simulink model "SCR_SiLS_R4_D102_test1"  (R2023a)
settings: Solver=VariableStepAuto  StartTime=0.0  StopTime=T_sim_end  RelTol=1e-3
model workspace (MAT data in the model file):
  ConnVar.ipAddress = '192.168.0.153'
  ConnVar.user = 'M1'
  ConnVar.pwd = [145 145 158 146 151 156 158 157]
  ConnVar.targetHandle = 0
libraries: M1SWBlocks x4
(part 1 of 2)
settings Model: Creator=CHSE  LastModifiedBy=gione
settings DebuggingCC: UnconnectedInputMsg=warning  UnconnectedOutputMsg=warning  UnconnectedLineMsg=warning
settings ModelReferenceCC: EnableRefExpFcnMdlSchedulingChecks=on
settings RTWCC: DLArmComputeVersion=19.05

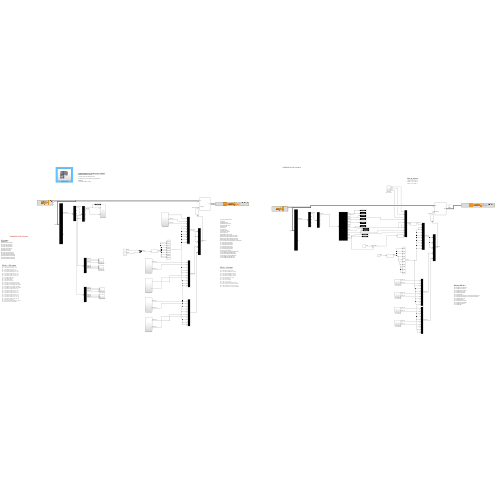
[thumbnail: Simulink's stored preview of the top-level diagram]
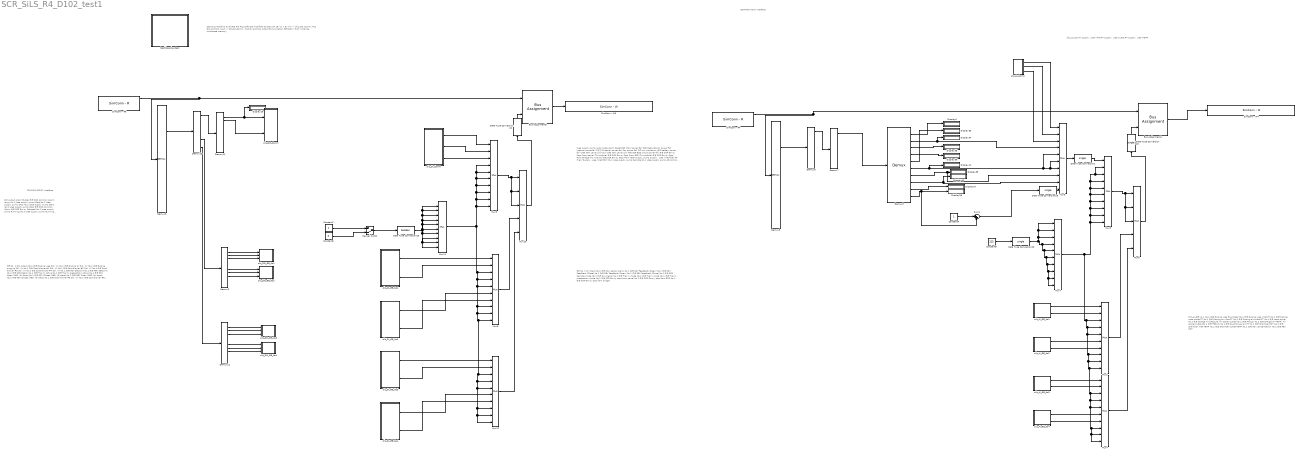
== system SCR_SiLS_R4_D102_test1 ==
  note: GE No. 1 DI intput
      |
      | No.1 G/E NOx sensor Alarm
      |
      | No.1 G/E RSV Feedback (Open)
      |
      | No.1 G/E RSV Feedback (Close)
      |
      | No.1 G/E RBV Feedback (Open)
      |
      | No.1 G/E RBV Feedback (Close)
      |
      | No.1 G/E SCR Remote mode
      |
      | No.1 G/E Run signal
      |
      | No.1 G/E Tier III mode
      |
      | No.1 G/E Tier II mode
      |
      | No.1 G/E Tier III preparation mode
      |
      | No.1 G/E SCR Em'cy stop from panel
      |
      | No.1 G/E SCR Emc'y stop from ECR
      |
      | No.1 G/E SCR Em'cy stop from bridge
  note: GE No. 1 DO output
      |
      | No.1 G/E Dosing urea Sol. VV
      |
      | No.1 G/E Dosing air Sol. VV
      |
      | No.1 G/E Dosing purging Sol. VV
      |
      | No.1 G/E Soot blower #1 Sol. VV
      |
      | No.1 G/E Soot blower #2 Sol. VV
      |
      | No.1 G/E Soot blower #3 Sol. VV
      |
      | No.1 G/E Soot blower #4 Sol. VV
      |
      | No.1 G/E RSV Setpoint
      |
      | No.1 G/E RBV Setpoint
      |
      | No.1 G/E SCR Ready
      |
      | No.1 G/E Tier III Active
      |
      | No.1 G/E Tier III preparation Active
      |
      | No.1 G/E RSV Open (ABS, NK class)
      |
      | No.1 G/E RSV Closed (ABS, NK class)
      |
      | No.1 G/E RBV Open (ABS, NK class)
      |
      | No.1 G/E RBV Closed (ABS, NK class)
      |
      | No.1 G/E Soot blower #5 Sol. VV
      |
      | No.1 G/E Soot blower #6 Sol. VV
      |
      | No.1 G/E Soot blower #7 Sol. VV
      |
      | No.1 G/E Soot blower #8 Sol. VV
      |
      | No.1 G/E Soot blower #9 Sol. VV
      |
      | No.1 G/E Soot blower #10 Sol. VV
      |
      | No.1 G/E Soot blower #11 Sol. VV
      |
      | No.1 G/E Soot blower #12 Sol. VV
      |
      | No.1 G/E Tier III Transfer
      |
      | No.1 SCR both bypass valve not open
      |
      | No.# G/E Common Shutdown
  note: DO output
      | Alarm Buzzer
      |
      | G/E SCR common alarm lamp
      |
      | No.1 Urea supply pump Start
      |
      | No.1 Urea supply pump Stop
      |
      | No.2 Urea supply pump Start
      |
      | No.2 Urea supply pump Stop
      |
      | G/E SCR common Alarm
      |
      | G/E SCR Em'cy Stopped
      |
      | No.1 Urea supply pump Running
      |
      | No.2 Urea supply pump Running
      |
      | No.1 G/E SCR Common Alarm lamp
      |
      | No.2 G/E SCR Common Alarm lamp
      |
      | No.3 G/E SCR Common Alarm lamp
      |
      | No.4 G/E SCR Common Alarm lamp
      |
      | ​
      |
      | ​
  note: Urea supply pump Auto mode
      |
      | Alarm Reset
      |
      | SCR Main power fail
      |
      | SCR Redundancy power fail
      |
      | Internal power fail(삭제됨)
      |
      | External power fail
      |
      | Fan power fail
      |
      | DC low insulation
      |
      | UPS battery power fail
      |
      | Urea tank Level Low-Low
      |
      | Urea tank Level Low
      |
      | G/E SCR ESD circuit power fail
      |
      | G/E SCR Em'cy Stop From panel (To module)
      |
      | G/E SCR Em'cy Stop From ECR (To module)
      |
      | G/E SCR Em'cy Stop From Bridge (To module)
      |
      | G/E SCR Em'cy Stop From Near Supply pump
      |
      | Supply, urea inlet filter dP High (Supply, urea inlet PDS)
      |
      | No.1 Urea supply pump Remote
      |
      | No.1 Urea supply pump Abnormal
      |
      | No.1 Urea supply pump Running
      |
      | No.2 Urea supply pump Remote
      |
      | No.2 Urea supply pump Abnormal
      |
      | No.2 Urea supply pump Running
      |
      | G/E Low Sulfur fuel supplied
      |
      | Urea tank drip tray Level High-High (ABS class)
      |
      | Urea tank TEMP High-High (ABS class)
      |
      | Urea tank Level High (ABS, BV, NK class)
      |
      | Urea tank drip tray Level High (ABS class)
      |
      | Urea tank TEMP Low (ABS, NK class)
      |
      | Urea tank TEMP High (ABS, NK class)
      |
      | ​
      |
      | ​
  note: COMMON DO/DI Interface
  note: SCR SiLS Model to evaluate the PLC software
      | modified at 2024.04.18. by Y.B. Kim
      |
      | -> Sils_DO_Comm: PLC DO and Sils input
      | -> Sils_DI_Comm : PLC DI and Sils output for simulation
      |
      | REMARK!!!
      | first, initialize workspace memory
  note: COMMON AO/AI Interface
  note: Sils_AI_Comm
      |
      | Supply, urea inlet PT
      |
      | Supply, urea outlet PT
      |
      | Supply, urea TEMP
  note: Sils_AI_GE no 1
      |
      | No.1 G/E Dosing urea flowmeter
      |
      | No.1 G/E Dosing urea inlet PT
      |
      | No.1 G/E Dosing urea outlet PT
      |
      | No.1 G/E Dosing air inlet PT
      |
      | No.1 G/E Dosing air outlet PT
      |
      | No.1 G/E Load signal
      |
      | No.1 G/E Charge Air pressure, Air cooler outlet (No.1 G/E PT212)
      |
      | No.1 G/E Charge Air TEMP, Air cooler outlet (No.1 G/E TE212)
      |
      | No.1 G/E Soot blower air PT
      |
      | No.1 G/E Chamber PDT
      |
      | No.1 G/E Chamber inlet TEMP
      |
      | No.1 G/E Chamber outlet TEMP
      |
      | No.1 G/E NOx concentration
      |
      | No.1 G/E RBV PDT
      |
      | ​
      |
      | ​
  Bus Assignment4 : BusAssignment  AssignedSignals=Moutput
  Bus Assignment5 : BusAssignment  AssignedSignals=Moutput
  Constant4 : Constant
  Constant5 : Constant  Value=123  VectorParams1D=off  OutDataTypeStr=single
  Constant6 : Constant  Value=0  VectorParams1D=off  OutDataTypeStr=boolean
  Constant7 : Constant  VectorParams1D=off  OutDataTypeStr=boolean
  Dashboard-system : Subsystem
  Data Type Conversion{1,18..20} (4 alike) : DataTypeConversion  OutDataTypeStr=single  SaturateOnIntegerOverflow=off  RndMeth=Floor
  Data Type Conversion22 : DataTypeConversion  OutDataTypeStr=boolean  SaturateOnIntegerOverflow=off  RndMeth=Floor
  Data Type Conversion23 : DataTypeConversion  OutDataTypeStr=boolean  SaturateOnIntegerOverflow=off  RndMeth=Floor
  Demux10 : Demux  Outputs=5
  Demux{2..3,7,11..12} (5 alike) : Demux  Outputs=10
  Demux5 : Demux  Outputs=2
  Demux6 : Demux  Outputs=5
  Demux9 : Demux  Outputs=2
  Display{6,18,33..41} (11 alike) : Display
      Display34 settings: Format=decimal (Stored Integer)
  Manual Switch : ManualSwitch  CurrentSetting=0
  Mux10 : Mux  Inputs=5
  Mux{2..5,7..9,11..12} (9 alike) : Mux  Inputs=10
      Mux11 settings: DisplayOption=signals
      Mux7 settings: DisplayOption=signals
  Mux6 : Mux  Inputs=5
  SimConn - R4 : M1SWBlocks/SimConn Blocks/SimConn - R  connVarName=ConnVar  InswModuleName='NONOXR4'  swModuleName=NONOXR4  InvarName='.gInterface.Analog'  varName=.gInterface.Analog  varDataType=Bus: Analog_typ  enRetOutput=on  enGetTrigger=off  getTrigger=rising  valDurLostConn=Zero  internalVal=0  DataDim=1  enSampTimMon=on  sampleTime=Ts_com
      settings: SourceProductName=Bachmann M1 Software
  SimConn - R5 : M1SWBlocks/SimConn Blocks/SimConn - R  connVarName=ConnVar  InswModuleName='NONOXR4'  swModuleName=NONOXR4  InvarName='.gInterface.Digital'  varName=.gInterface.Digital  varDataType=Bus: Digital_typ  enRetOutput=on  enGetTrigger=off  getTrigger=rising  valDurLostConn=Zero  internalVal=0  DataDim=1  enSampTimMon=on  sampleTime=Ts_com
      settings: SourceProductName=Bachmann M1 Software
  SimConn - W4 : M1SWBlocks/SimConn Blocks/SimConn - W  connVarName=ConnVar  InswModuleName='NONOXR4'  swModuleName=NONOXR4  InvarName='.gInterface.Analog'  varName=.gInterface.Analog  varDataType=Bus: Analog_typ  enRetOutput=off  enGetTrigger=off  getTrigger=rising  enSampTimMon=on
      settings: SourceProductName=Bachmann M1 Software
  SimConn - W5 : M1SWBlocks/SimConn Blocks/SimConn - W  connVarName=ConnVar  InswModuleName='NONOXR4'  swModuleName=NONOXR4  InvarName='.gInterface.Digital'  varName=.gInterface.Digital  varDataType=Bus: Digital_typ  enRetOutput=off  enGetTrigger=off  getTrigger=rising  enSampTimMon=off
      settings: SourceProductName=Bachmann M1 Software
  Sum4 : Sum  Inputs=|++
  sils_AI_Comm : Subsystem
  sils_AI_GE_No1 : Subsystem
  sils_AI_GE_No2 : Subsystem
  sils_AI_GE_No3 : Subsystem
  sils_AI_GE_No4 : Subsystem
  sils_DI_Comm : Subsystem
  sils_DI_GE_No1 : Subsystem
  sils_DI_GE_No2 : Subsystem
  sils_DI_GE_No3 : Subsystem
  sils_DI_GE_No4 : Subsystem
  sils_DO_Comm : Subsystem
  sils_DO_GE_No1 : Subsystem
  sils_DO_GE_No2 : Subsystem
  sils_DO_GE_No3 : Subsystem
  sils_DO_GE_No4 : Subsystem
  wires:
  Demux11/1 -> sils_DO_Comm/1(In1), Display18/1
  sils_DI_Comm/1(Out2) -> Mux9/1
  sils_DI_Comm/2(Out3) -> Mux9/2
  Mux3/1 -> Data Type Conversion1/1
  Demux3/3 -> Display35/1
  Data Type Conversion18/1 -> Mux3/10
  Demux3/7 -> Mux3/8, Display39/1
  Demux3/6 -> Mux3/5, Mux3/6, Mux3/7, Display41/1
  Demux3/8 -> Mux3/9, Display40/1
  Constant4/1 -> Sum4/1
  Sum4/1 -> Data Type Conversion18/1
  SimConn - R4/1 -> Bus Assignment4/1, Demux5/1
  Demux3/1 -> Display6/1
  Demux3/10 -> Sum4/2, Display38/1
  Demux3/9 -> Display37/1
  Demux3/4 -> Display36/1
  Bus Assignment4/1 -> SimConn - W4/1
  Demux5/1 -> Demux6/1
  Demux6/1 -> Demux7/1
  Demux7/1 -> Demux3/1
  Mux5/1 -> Mux6/3, Mux6/2, Mux6/1
  Mux6/1 -> Data Type Conversion19/1
  Demux3/2 -> Mux3/4, Display34/1
  Demux3/5 -> Display33/1
  Constant5/1 -> Data Type Conversion20/1
  Mux7/1 -> Mux4/10, Mux4/9, Mux4/8, Mux4/5, Mux4/4, Mux4/3, Mux2/10, Mux2/9, Mux2/8, Mux2/5, Mux2/4, Mux2/3, Mux5/10, Mux5/9, Mux5/8, Mux5/7, Mux5/6, Mux5/5, Mux5/4, Mux5/2, Mux5/3
  Data Type Conversion19/1 -> Bus Assignment4/2
  Data Type Conversion20/1 -> Mux7/3, Mux7/2, Mux7/1, Mux7/10, Mux7/9, Mux7/8, Mux7/7, Mux7/6, Mux7/5, Mux7/4
  Constant7/1 -> Manual Switch/1
  Data Type Conversion22/1 -> Bus Assignment5/2
  Demux10/1 -> Demux11/1
  Mux9/1 -> Mux10/3, Mux10/2, Mux10/1
  Mux10/1 -> Data Type Conversion22/1
  Data Type Conversion23/1 -> Mux11/3, Mux11/1, Mux11/2, Mux11/4, Mux11/8, Mux11/10, Mux11/9, Mux11/7, Mux11/6, Mux11/5
  Bus Assignment5/1 -> SimConn - W5/1
  SimConn - R5/1 -> Bus Assignment5/1, Demux9/1
  Demux9/1 -> Demux10/1
  Constant6/1 -> Manual Switch/2
  Manual Switch/1 -> Data Type Conversion23/1
  Demux11/2 -> sils_DO_Comm/2(In2)
  sils_DI_Comm/3(Out1) -> Mux9/3
  sils_DI_GE_No1/1(Out2) -> Mux8/1
  sils_DI_GE_No1/2(Out1) -> Mux8/2
  Mux8/1 -> Mux10/4
  sils_DI_GE_No2/1(Out2) -> Mux8/6
  sils_DI_GE_No2/2(Out1) -> Mux8/7
  Mux11/1 -> Mux9/10, Mux9/9, Mux9/8, Mux9/7, Mux9/6, Mux9/5, Mux9/4, Mux12/10, Mux12/9, Mux12/8, Mux12/5, Mux12/4, Mux12/3, Mux8/10, Mux8/9, Mux8/8, Mux8/5, Mux8/4, Mux8/3
  sils_DI_GE_No3/2(Out1) -> Mux12/2
  Mux12/1 -> Mux10/5
  sils_DI_GE_No3/1(Out2) -> Mux12/1
  sils_DI_GE_No4/2(Out1) -> Mux12/7
  sils_DI_GE_No4/1(Out2) -> Mux12/6
  Demux10/4 -> Demux2/1
  Demux2/1 -> sils_DO_GE_No1/1(In1)
  Demux2/2 -> sils_DO_GE_No1/2(In2)
  Demux10/5 -> Demux12/1
  sils_AI_Comm/1(Out1) -> Mux3/1
  sils_AI_Comm/2(Out2) -> Mux3/2
  sils_AI_Comm/3(Out3) -> Mux3/3
  sils_AI_GE_No1/1(Out1) -> Mux2/1
  sils_AI_GE_No1/2(Out2) -> Mux2/2
  Mux2/1 -> Mux6/4
  sils_AI_GE_No2/1(Out1) -> Mux2/6
  sils_AI_GE_No2/2(Out2) -> Mux2/7
  sils_AI_GE_No4/1(Out1) -> Mux4/6
  sils_AI_GE_No3/2(Out2) -> Mux4/2
  sils_AI_GE_No3/1(Out1) -> Mux4/1
  sils_AI_GE_No4/2(Out2) -> Mux4/7
  Mux4/1 -> Mux6/5
  Data Type Conversion1/1 -> Mux5/1
  Demux2/3 -> sils_DO_GE_No1/3(In3)
  Demux12/1 -> sils_DO_GE_No3/1(In1)
  Demux12/2 -> sils_DO_GE_No3/2(In2)
  Demux12/3 -> sils_DO_GE_No3/3(In3)
  Demux2/6 -> sils_DO_GE_No2/1(In1)
  Demux2/7 -> sils_DO_GE_No2/2(In2)
  Demux2/8 -> sils_DO_GE_No2/3(In3)
  Demux12/6 -> sils_DO_GE_No4/1(In1)
  Demux12/8 -> sils_DO_GE_No4/3(In3)
  Demux12/7 -> sils_DO_GE_No4/2(In2)

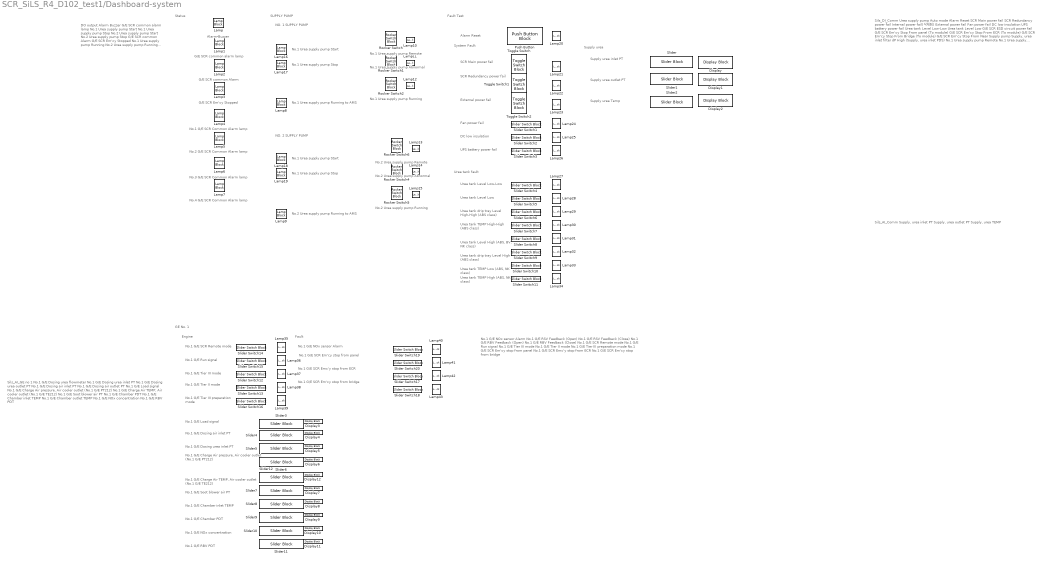
== system SCR_SiLS_R4_D102_test1/Dashboard-system ==
  note: Fault
  note: Engine
  note: GE No. 1
  note: Supply urea
  note: Urea tank fault
  note: System Fault
  note: NO. 1 SUPPLY PUMP
  note: SUPPLY PUMP
  note: Alarm Buzzer
  note: G/E SCR common alarm lamp
  note: DO output
      | Alarm Buzzer
      |
      | G/E SCR common alarm lamp
      |
      | No.1 Urea supply pump Start
      |
      | No.1 Urea supply pump Stop
      |
      | No.2 Urea supply pump Start
      |
      | No.2 Urea supply pump Stop
      |
      | G/E SCR common Alarm
      |
      | G/E SCR Em'cy Stopped
      |
      | No.1 Urea supply pump Running
      |
      | No.2 Urea supply pump Running
      |
      | No.1 G/E SCR Common Alarm lamp
      |
      | No.2 G/E SCR Common Alarm lamp
      |
      | No.3 G/E SCR Common Alarm lamp
      |
      | No.4 G/E SCR Common Alarm lamp
      |
      | ​
      |
      | ​
  note: G/E SCR Em'cy Stopped
  note: G/E SCR common Alarm
  note: No.1 G/E SCR Common Alarm lamp
  note: No.2 G/E SCR Common Alarm lamp
  note: No.3 G/E SCR Common Alarm lamp
  note: No.4 G/E SCR Common Alarm lamp
  note: Status
  note: No.1 Urea supply pump Running to AMS
  note: NO. 2 SUPPLY PUMP
  note: No.2 Urea supply pump Running to AMS
  note: No.1 Urea supply pump Remote
  note: No.1 Urea supply pump Abnormal
  note: No.1 Urea supply pump Running
  note: Sils_DI_Comm
      |
      | Urea supply pump Auto mode
      |
      | Alarm Reset
      |
      | SCR Main power fail
      |
      | SCR Redundancy power fail
      |
      | Internal power fail(삭제됨)
      |
      | External power fail
      |
      | Fan power fail
      |
      | DC low insulation
      |
      | UPS battery power fail
      |
      | Urea tank Level Low-Low
      |
      | Urea tank Level Low
      |
      | G/E SCR ESD circuit power fail
      |
      | G/E SCR Em'cy Stop From panel (To module)
      |
      | G/E SCR Em'cy Stop From ECR (To module)
      |
      | G/E SCR Em'cy Stop From Bridge (To module)
      |
      | G/E SCR Em'cy Stop From Near Supply pump
      |
      | Supply, urea inlet filter dP High (Supply, urea inlet PDS)
      |
      | No.1 Urea supply pump Remote
      |
      | No.1 Urea supply pump Abnormal
      |
      | No.1 Urea supply pump Running
      |
      | No.2 Urea supply pump Remote
      |
      | No.2 Urea supply pump Abnormal
      |
      | No.2 Urea supply pump Running
      |
      | G/E Low Sulfur fuel supplied
      |
      | Urea tank drip tray Level High-High (ABS class)
      |
      | Urea tank TEMP High-High (ABS class)
      |
      | Urea tank Level High (ABS, BV, NK class)
      |
      | Urea tank drip tray Level High (ABS class)
      |
      | Urea tank TEMP Low (ABS, NK class)
      |
      | Urea tank TEMP High (ABS, NK class)
      |
      | ​
      |
      | ​
  note: No.2 Urea supply pump Running
  note: No.2 Urea supply pump Abnormal
  note: No.2 Urea supply pump Remote
  note: No.1 Urea supply pump Start
  note: No.1 Urea supply pump Stop
  note: No.1 Urea supply pump Stop
  note: No.1 Urea supply pump Start
  note: Fault Test
  note: Alarm Reset
  note: SCR Main power fail
  note: SCR Redundancy power fail
  note: External power fail
  note: Fan power fail
  note: DC low insulation
  note: UPS battery power fail
  note: Urea tank Level Low-Low
  note: Urea tank Level Low
  note: Urea tank drip tray Level High-High (ABS class)
  note: Urea tank TEMP High-High (ABS class)
  note: Urea tank Level High (ABS, BV, NK class)
  note: Urea tank drip tray Level High (ABS class)
  note: Urea tank TEMP Low (ABS, NK class)
  note: Urea tank TEMP High (ABS, NK class)
  note: Supply urea inlet PT
  note: Sils_AI_Comm
      |
      | Supply, urea inlet PT
      |
      | Supply, urea outlet PT
      |
      | Supply, urea TEMP
  note: Supply urea outlet PT
  note: Supply urea Temp
  note: No.1 G/E NOx sensor Alarm
      |
      | No.1 G/E RSV Feedback (Open)
      |
      | No.1 G/E RSV Feedback (Close)
      |
      | No.1 G/E RBV Feedback (Open)
      |
      | No.1 G/E RBV Feedback (Close)
      |
      | No.1 G/E SCR Remote mode
      |
      | No.1 G/E Run signal
      |
      | No.1 G/E Tier III mode
      |
      | No.1 G/E Tier II mode
      |
      | No.1 G/E Tier III preparation mode
      |
      | No.1 G/E SCR Em'cy stop from panel
      |
      | No.1 G/E SCR Emc'y stop from ECR
      |
      | No.1 G/E SCR Em'cy stop from bridge
  note: No.1 G/E Tier II mode
  note: No.1 G/E Tier III mode
  note: No.1 G/E Run signal
  note: No.1 G/E SCR Remote mode
  note: No.1 G/E Tier III preparation mode
  note: No.1 G/E SCR Emc'y stop from ECR
  note: No.1 G/E SCR Em'cy stop from bridge
  note: No.1 G/E NOx sensor Alarm
  note: No.1 G/E SCR Em'cy stop from panel
  note: No.1 G/E Load signal
  note: Sils_AI_GE no 1
      |
      | No.1 G/E Dosing urea flowmeter
      |
      | No.1 G/E Dosing urea inlet PT
      |
      | No.1 G/E Dosing urea outlet PT
      |
      | No.1 G/E Dosing air inlet PT
      |
      | No.1 G/E Dosing air outlet PT
      |
      | No.1 G/E Load signal
      |
      | No.1 G/E Charge Air pressure, Air cooler outlet (No.1 G/E PT212)
      |
      | No.1 G/E Charge Air TEMP, Air cooler outlet (No.1 G/E TE212)
      |
      | No.1 G/E Soot blower air PT
      |
      | No.1 G/E Chamber PDT
      |
      | No.1 G/E Chamber inlet TEMP
      |
      | No.1 G/E Chamber outlet TEMP
      |
      | No.1 G/E NOx concentration
      |
      | No.1 G/E RBV PDT
      |
      | ​
      |
      | ​
  note: No.1 G/E Dosing air inlet PT
  note: No.1 G/E Dosing urea inlet PT
  note: No.1 G/E Charge Air pressure, Air cooler outlet (No.1 G/E PT212)
  note: No.1 G/E Soot blower air PT
  note: No.1 G/E Chamber inlet TEMP
  note: No.1 G/E Chamber PDT
  note: No.1 G/E NOx concentration
  note: No.1 G/E RBV PDT
  note: No.1 G/E Charge Air TEMP, Air cooler outlet (No.1 G/E TE212)
  Display{,1..12} (13 alike) : DisplayBlock  LabelPosition=Hide  Transparency=1
  Lamp{,1..43} (44 alike) : LampBlock  LabelPosition=Hide
  Push Button : PushButtonBlock  ButtonText=Alarm Reset  OffValue=0.000000
  Rocker Switch{,1..2,4..6} (6 alike) : RockerSwitchBlock  LabelPosition=Hide
      settings: Values={{'Off', 'On'}, [0 1]}
  Slider : SliderBlock  LabelPosition=Hide  ScaleMax=16
  Slider Switch{1..20} (20 alike) : SliderSwitchBlock  LabelPosition=Hide
      settings: Values={{'Off', 'On'}, [0 1]}
  Slider1 : SliderBlock  LabelPosition=Hide  ScaleMax=16
  Slider10 : SliderBlock  LabelPosition=Hide  ScaleMax=120
  Slider11 : SliderBlock  LabelPosition=Hide
  Slider12 : SliderBlock  LabelPosition=Hide  ScaleMax=200
  Slider2 : SliderBlock  LabelPosition=Hide
  Slider3 : SliderBlock  LabelPosition=Hide  ScaleMax=120
  Slider4 : SliderBlock  LabelPosition=Hide  ScaleMax=15
  Slider5 : SliderBlock  LabelPosition=Hide  ScaleMax=15
  Slider6 : SliderBlock  LabelPosition=Hide  ScaleMax=10
  Slider7 : SliderBlock  LabelPosition=Hide  ScaleMax=120
  Slider8 : SliderBlock  LabelPosition=Hide  ScaleMax=600
  Slider9 : SliderBlock  LabelPosition=Hide
  Toggle Switch : ToggleSwitchBlock  LabelPosition=Hide
      settings: Values={{'Off', 'On'}, [0 1]}
  Toggle Switch1 : ToggleSwitchBlock  LabelPosition=Hide
      settings: Values={{'Off', 'On'}, [0 1]}
  Toggle Switch2 : ToggleSwitchBlock  LabelPosition=Hide
      settings: Values={{'Off', 'On'}, [0 1]}

== system SCR_SiLS_R4_D102_test1/sils_AI_Comm ==
  note: Sils_AI_Comm
      |
      | Supply, urea inlet PT
      |
      | Supply, urea outlet PT
      |
      | Supply, urea TEMP
  Data Type Conversion3 : DataTypeConversion  OutDataTypeStr=single  SaturateOnIntegerOverflow=off  RndMeth=Floor
  Data Type Conversion4 : DataTypeConversion  OutDataTypeStr=single  SaturateOnIntegerOverflow=off  RndMeth=Floor
  Data Type Conversion7 : DataTypeConversion  OutDataTypeStr=single  SaturateOnIntegerOverflow=off  RndMeth=Floor
  Gain : Gain  Gain=1.0
  Gain1 : Gain
  Gain2 : Gain
  Supply urea TEMP : Constant  Value=26
  Supply urea inlet PT : Constant  Value=4
  Supply urea outlet PT : Constant  Value=7
  Out1 : Outport
  Out2 : Outport  Port=2
  Out3 : Outport  Port=3
  wires:
  Supply urea inlet PT/1 -> Gain/1
  Supply urea outlet PT/1 -> Gain1/1
  Gain1/1 -> Data Type Conversion3/1
  Data Type Conversion3/1 -> Out2/1
  Supply urea TEMP/1 -> Gain2/1
  Gain2/1 -> Data Type Conversion4/1
  Gain/1 -> Data Type Conversion7/1
  Data Type Conversion7/1 -> Out1/1
  Data Type Conversion4/1 -> Out3/1

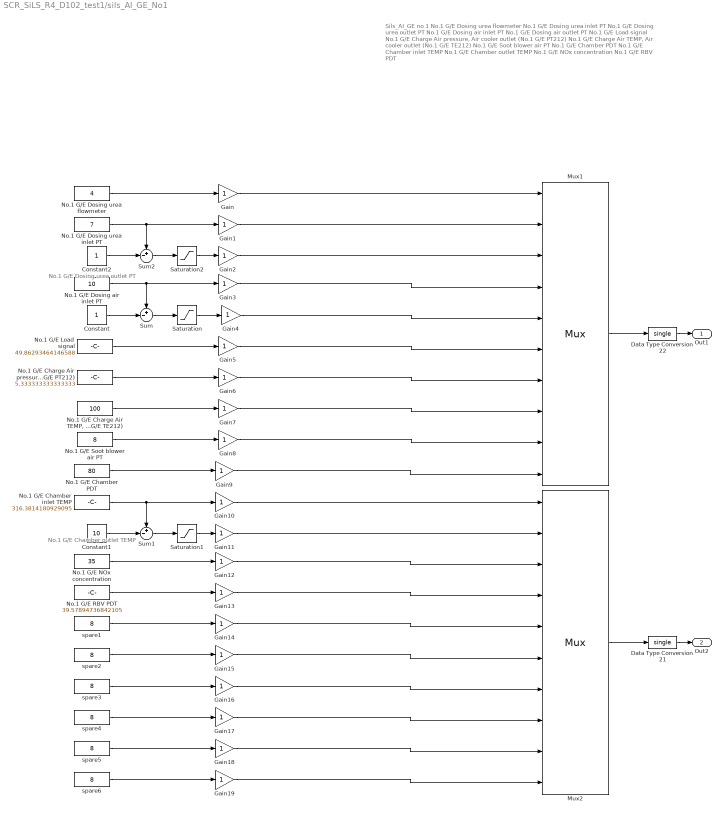
== system SCR_SiLS_R4_D102_test1/sils_AI_GE_No1 ==
  note: No.1 G/E Dosing urea outlet PT
  note: No.1 G/E Chamber outlet TEMP
  note: Sils_AI_GE no 1
      |
      | No.1 G/E Dosing urea flowmeter
      |
      | No.1 G/E Dosing urea inlet PT
      |
      | No.1 G/E Dosing urea outlet PT
      |
      | No.1 G/E Dosing air inlet PT
      |
      | No.1 G/E Dosing air outlet PT
      |
      | No.1 G/E Load signal
      |
      | No.1 G/E Charge Air pressure, Air cooler outlet (No.1 G/E PT212)
      |
      | No.1 G/E Charge Air TEMP, Air cooler outlet (No.1 G/E TE212)
      |
      | No.1 G/E Soot blower air PT
      |
      | No.1 G/E Chamber PDT
      |
      | No.1 G/E Chamber inlet TEMP
      |
      | No.1 G/E Chamber outlet TEMP
      |
      | No.1 G/E NOx concentration
      |
      | No.1 G/E RBV PDT
      |
      | ​
      |
      | ​
  Constant : Constant
  Constant1 : Constant  Value=10
  Constant2 : Constant
  Data Type Conversion21 : DataTypeConversion  OutDataTypeStr=single  SaturateOnIntegerOverflow=off  RndMeth=Floor
  Data Type Conversion22 : DataTypeConversion  OutDataTypeStr=single  SaturateOnIntegerOverflow=off  RndMeth=Floor
  Gain{,1..19} (20 alike) : Gain
  Mux1 : Mux  Inputs=10
  Mux2 : Mux  Inputs=10
  No.1 G/E Chamber PDT : Constant  Value=80
  No.1 G/E Chamber inlet TEMP : Constant  Value=316.3814180929095
  "No.1 G/E Charge Air TEMP, Air cooler outlet (No.1 G/E TE212)" : Constant  Value=100
  "No.1 G/E Charge Air pressure, Air cooler outlet (No.1 G/E PT212)" : Constant  Value=5.333333333333333
  No.1 G/E Dosing air inlet PT : Constant  Value=10
  No.1 G/E Dosing urea flowmeter : Constant  Value=4
  No.1 G/E Dosing urea inlet PT : Constant  Value=7
  No.1 G/E Load signal : Constant  Value=49.86293464146588
  No.1 G/E NOx concentration : Constant  Value=35
  No.1 G/E RBV PDT : Constant  Value=39.57894736842105
  No.1 G/E Soot blower air PT : Constant  Value=8
  Saturation : Saturate  UpperLimit=10.0  LowerLimit=0.0
  Saturation1 : Saturate  UpperLimit=500.0  LowerLimit=0.0
  Saturation2 : Saturate  UpperLimit=10.0  LowerLimit=0.0
  Sum : Sum  Inputs=+-|
  Sum1 : Sum  Inputs=+-|
  Sum2 : Sum  Inputs=+-|
  spare{1..6} (6 alike) : Constant  Value=8
  Out1 : Outport
  Out2 : Outport  Port=2
  wires:
  No.1 G/E Dosing urea flowmeter/1 -> Gain/1
  Gain1/1 -> Mux1/2
  Gain/1 -> Mux1/1
  Gain2/1 -> Mux1/3
  No.1 G/E Dosing air inlet PT/1 -> Gain3/1, Sum/1
  Sum/1 -> Saturation/1
  No.1 G/E Load signal/1 -> Gain5/1
  Gain3/1 -> Mux1/4
  Gain4/1 -> Mux1/5
  Gain5/1 -> Mux1/6
  "No.1 G/E Charge Air pressure, Air cooler outlet (No.1 G/E PT212)"/1 -> Gain6/1
  "No.1 G/E Charge Air TEMP, Air cooler outlet (No.1 G/E TE212)"/1 -> Gain7/1
  No.1 G/E Soot blower air PT/1 -> Gain8/1
  Gain6/1 -> Mux1/7
  Gain7/1 -> Mux1/8
  Gain8/1 -> Mux1/9
  No.1 G/E Chamber PDT/1 -> Gain9/1
  No.1 G/E Chamber inlet TEMP/1 -> Sum1/1, Gain10/1
  Gain9/1 -> Mux1/10
  Gain10/1 -> Mux2/1
  Gain11/1 -> Mux2/2
  No.1 G/E RBV PDT/1 -> Gain13/1
  Gain13/1 -> Mux2/4
  Gain12/1 -> Mux2/3
  No.1 G/E NOx concentration/1 -> Gain12/1
  Constant/1 -> Sum/2
  Saturation/1 -> Gain4/1
  Sum1/1 -> Saturation1/1
  Constant1/1 -> Sum1/2
  Saturation1/1 -> Gain11/1
  No.1 G/E Dosing urea inlet PT/1 -> Gain1/1, Sum2/1
  Sum2/1 -> Saturation2/1
  Constant2/1 -> Sum2/2
  Saturation2/1 -> Gain2/1
  spare1/1 -> Gain14/1
  Gain14/1 -> Mux2/5
  spare2/1 -> Gain15/1
  Gain15/1 -> Mux2/6
  spare3/1 -> Gain16/1
  Gain16/1 -> Mux2/7
  spare4/1 -> Gain17/1
  Gain17/1 -> Mux2/8
  spare5/1 -> Gain18/1
  Gain18/1 -> Mux2/9
  spare6/1 -> Gain19/1
  Gain19/1 -> Mux2/10
  Mux1/1 -> Data Type Conversion22/1
  Mux2/1 -> Data Type Conversion21/1
  Data Type Conversion21/1 -> Out2/1
  Data Type Conversion22/1 -> Out1/1

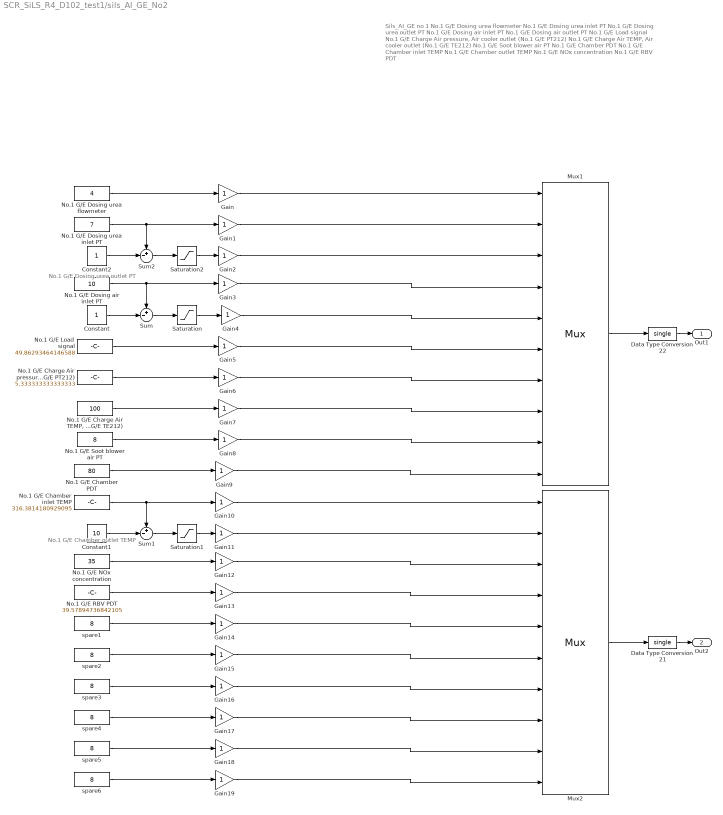
== system SCR_SiLS_R4_D102_test1/sils_AI_GE_No2 ==
  note: No.1 G/E Dosing urea outlet PT
  note: No.1 G/E Chamber outlet TEMP
  note: Sils_AI_GE no 1
      |
      | No.1 G/E Dosing urea flowmeter
      |
      | No.1 G/E Dosing urea inlet PT
      |
      | No.1 G/E Dosing urea outlet PT
      |
      | No.1 G/E Dosing air inlet PT
      |
      | No.1 G/E Dosing air outlet PT
      |
      | No.1 G/E Load signal
      |
      | No.1 G/E Charge Air pressure, Air cooler outlet (No.1 G/E PT212)
      |
      | No.1 G/E Charge Air TEMP, Air cooler outlet (No.1 G/E TE212)
      |
      | No.1 G/E Soot blower air PT
      |
      | No.1 G/E Chamber PDT
      |
      | No.1 G/E Chamber inlet TEMP
      |
      | No.1 G/E Chamber outlet TEMP
      |
      | No.1 G/E NOx concentration
      |
      | No.1 G/E RBV PDT
      |
      | ​
      |
      | ​
  Constant : Constant
  Constant1 : Constant  Value=10
  Constant2 : Constant
  Data Type Conversion21 : DataTypeConversion  OutDataTypeStr=single  SaturateOnIntegerOverflow=off  RndMeth=Floor
  Data Type Conversion22 : DataTypeConversion  OutDataTypeStr=single  SaturateOnIntegerOverflow=off  RndMeth=Floor
  Gain{,1..19} (20 alike) : Gain
  Mux1 : Mux  Inputs=10
  Mux2 : Mux  Inputs=10
  No.1 G/E Chamber PDT : Constant  Value=80
  No.1 G/E Chamber inlet TEMP : Constant  Value=316.3814180929095
  "No.1 G/E Charge Air TEMP, Air cooler outlet (No.1 G/E TE212)" : Constant  Value=100
  "No.1 G/E Charge Air pressure, Air cooler outlet (No.1 G/E PT212)" : Constant  Value=5.333333333333333
  No.1 G/E Dosing air inlet PT : Constant  Value=10
  No.1 G/E Dosing urea flowmeter : Constant  Value=4
  No.1 G/E Dosing urea inlet PT : Constant  Value=7
  No.1 G/E Load signal : Constant  Value=49.86293464146588
  No.1 G/E NOx concentration : Constant  Value=35
  No.1 G/E RBV PDT : Constant  Value=39.57894736842105
  No.1 G/E Soot blower air PT : Constant  Value=8
  Saturation : Saturate  UpperLimit=10.0  LowerLimit=0.0
  Saturation1 : Saturate  UpperLimit=500.0  LowerLimit=0.0
  Saturation2 : Saturate  UpperLimit=10.0  LowerLimit=0.0
  Sum : Sum  Inputs=+-|
  Sum1 : Sum  Inputs=+-|
  Sum2 : Sum  Inputs=+-|
  spare{1..6} (6 alike) : Constant  Value=8
  Out1 : Outport
  Out2 : Outport  Port=2
  wires:
  No.1 G/E Dosing urea flowmeter/1 -> Gain/1
  Gain1/1 -> Mux1/2
  Gain/1 -> Mux1/1
  Gain2/1 -> Mux1/3
  No.1 G/E Dosing air inlet PT/1 -> Gain3/1, Sum/1
  Sum/1 -> Saturation/1
  No.1 G/E Load signal/1 -> Gain5/1
  Gain3/1 -> Mux1/4
  Gain4/1 -> Mux1/5
  Gain5/1 -> Mux1/6
  "No.1 G/E Charge Air pressure, Air cooler outlet (No.1 G/E PT212)"/1 -> Gain6/1
  "No.1 G/E Charge Air TEMP, Air cooler outlet (No.1 G/E TE212)"/1 -> Gain7/1
  No.1 G/E Soot blower air PT/1 -> Gain8/1
  Gain6/1 -> Mux1/7
  Gain7/1 -> Mux1/8
  Gain8/1 -> Mux1/9
  No.1 G/E Chamber PDT/1 -> Gain9/1
  No.1 G/E Chamber inlet TEMP/1 -> Sum1/1, Gain10/1
  Gain9/1 -> Mux1/10
  Gain10/1 -> Mux2/1
  Gain11/1 -> Mux2/2
  No.1 G/E RBV PDT/1 -> Gain13/1
  Gain13/1 -> Mux2/4
  Gain12/1 -> Mux2/3
  No.1 G/E NOx concentration/1 -> Gain12/1
  Constant/1 -> Sum/2
  Saturation/1 -> Gain4/1
  Sum1/1 -> Saturation1/1
  Constant1/1 -> Sum1/2
  Saturation1/1 -> Gain11/1
  No.1 G/E Dosing urea inlet PT/1 -> Gain1/1, Sum2/1
  Sum2/1 -> Saturation2/1
  Constant2/1 -> Sum2/2
  Saturation2/1 -> Gain2/1
  spare1/1 -> Gain14/1
  Gain14/1 -> Mux2/5
  spare2/1 -> Gain15/1
  Gain15/1 -> Mux2/6
  spare3/1 -> Gain16/1
  Gain16/1 -> Mux2/7
  spare4/1 -> Gain17/1
  Gain17/1 -> Mux2/8
  spare5/1 -> Gain18/1
  Gain18/1 -> Mux2/9
  spare6/1 -> Gain19/1
  Gain19/1 -> Mux2/10
  Mux1/1 -> Data Type Conversion22/1
  Mux2/1 -> Data Type Conversion21/1
  Data Type Conversion21/1 -> Out2/1
  Data Type Conversion22/1 -> Out1/1

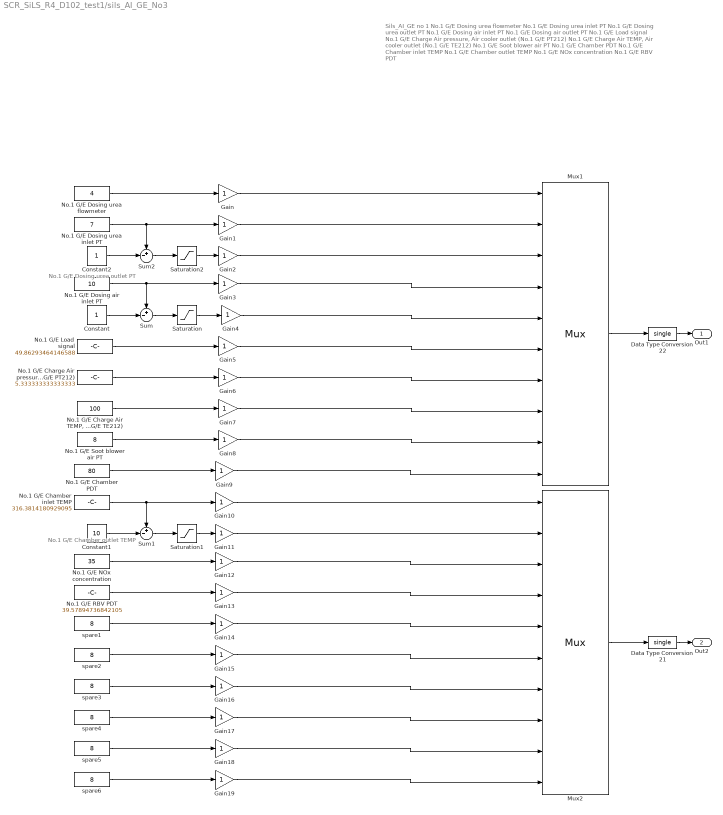
== system SCR_SiLS_R4_D102_test1/sils_AI_GE_No3 ==
  note: No.1 G/E Dosing urea outlet PT
  note: No.1 G/E Chamber outlet TEMP
  note: Sils_AI_GE no 1
      |
      | No.1 G/E Dosing urea flowmeter
      |
      | No.1 G/E Dosing urea inlet PT
      |
      | No.1 G/E Dosing urea outlet PT
      |
      | No.1 G/E Dosing air inlet PT
      |
      | No.1 G/E Dosing air outlet PT
      |
      | No.1 G/E Load signal
      |
      | No.1 G/E Charge Air pressure, Air cooler outlet (No.1 G/E PT212)
      |
      | No.1 G/E Charge Air TEMP, Air cooler outlet (No.1 G/E TE212)
      |
      | No.1 G/E Soot blower air PT
      |
      | No.1 G/E Chamber PDT
      |
      | No.1 G/E Chamber inlet TEMP
      |
      | No.1 G/E Chamber outlet TEMP
      |
      | No.1 G/E NOx concentration
      |
      | No.1 G/E RBV PDT
      |
      | ​
      |
      | ​
  Constant : Constant
  Constant1 : Constant  Value=10
  Constant2 : Constant
  Data Type Conversion21 : DataTypeConversion  OutDataTypeStr=single  SaturateOnIntegerOverflow=off  RndMeth=Floor
  Data Type Conversion22 : DataTypeConversion  OutDataTypeStr=single  SaturateOnIntegerOverflow=off  RndMeth=Floor
  Gain{,1..19} (20 alike) : Gain
  Mux1 : Mux  Inputs=10
  Mux2 : Mux  Inputs=10
  No.1 G/E Chamber PDT : Constant  Value=80
  No.1 G/E Chamber inlet TEMP : Constant  Value=316.3814180929095
  "No.1 G/E Charge Air TEMP, Air cooler outlet (No.1 G/E TE212)" : Constant  Value=100
  "No.1 G/E Charge Air pressure, Air cooler outlet (No.1 G/E PT212)" : Constant  Value=5.333333333333333
  No.1 G/E Dosing air inlet PT : Constant  Value=10
  No.1 G/E Dosing urea flowmeter : Constant  Value=4
  No.1 G/E Dosing urea inlet PT : Constant  Value=7
  No.1 G/E Load signal : Constant  Value=49.86293464146588
  No.1 G/E NOx concentration : Constant  Value=35
  No.1 G/E RBV PDT : Constant  Value=39.57894736842105
  No.1 G/E Soot blower air PT : Constant  Value=8
  Saturation : Saturate  UpperLimit=10.0  LowerLimit=0.0
  Saturation1 : Saturate  UpperLimit=500.0  LowerLimit=0.0
  Saturation2 : Saturate  UpperLimit=10.0  LowerLimit=0.0
  Sum : Sum  Inputs=+-|
  Sum1 : Sum  Inputs=+-|
  Sum2 : Sum  Inputs=+-|
  spare{1..6} (6 alike) : Constant  Value=8
  Out1 : Outport
  Out2 : Outport  Port=2
  wires:
  No.1 G/E Dosing urea flowmeter/1 -> Gain/1
  Gain1/1 -> Mux1/2
  Gain/1 -> Mux1/1
  Gain2/1 -> Mux1/3
  No.1 G/E Dosing air inlet PT/1 -> Gain3/1, Sum/1
  Sum/1 -> Saturation/1
  No.1 G/E Load signal/1 -> Gain5/1
  Gain3/1 -> Mux1/4
  Gain4/1 -> Mux1/5
  Gain5/1 -> Mux1/6
  "No.1 G/E Charge Air pressure, Air cooler outlet (No.1 G/E PT212)"/1 -> Gain6/1
  "No.1 G/E Charge Air TEMP, Air cooler outlet (No.1 G/E TE212)"/1 -> Gain7/1
  No.1 G/E Soot blower air PT/1 -> Gain8/1
  Gain6/1 -> Mux1/7
  Gain7/1 -> Mux1/8
  Gain8/1 -> Mux1/9
  No.1 G/E Chamber PDT/1 -> Gain9/1
  No.1 G/E Chamber inlet TEMP/1 -> Sum1/1, Gain10/1
  Gain9/1 -> Mux1/10
  Gain10/1 -> Mux2/1
  Gain11/1 -> Mux2/2
  No.1 G/E RBV PDT/1 -> Gain13/1
  Gain13/1 -> Mux2/4
  Gain12/1 -> Mux2/3
  No.1 G/E NOx concentration/1 -> Gain12/1
  Constant/1 -> Sum/2
  Saturation/1 -> Gain4/1
  Sum1/1 -> Saturation1/1
  Constant1/1 -> Sum1/2
  Saturation1/1 -> Gain11/1
  No.1 G/E Dosing urea inlet PT/1 -> Gain1/1, Sum2/1
  Sum2/1 -> Saturation2/1
  Constant2/1 -> Sum2/2
  Saturation2/1 -> Gain2/1
  spare1/1 -> Gain14/1
  Gain14/1 -> Mux2/5
  spare2/1 -> Gain15/1
  Gain15/1 -> Mux2/6
  spare3/1 -> Gain16/1
  Gain16/1 -> Mux2/7
  spare4/1 -> Gain17/1
  Gain17/1 -> Mux2/8
  spare5/1 -> Gain18/1
  Gain18/1 -> Mux2/9
  spare6/1 -> Gain19/1
  Gain19/1 -> Mux2/10
  Mux1/1 -> Data Type Conversion22/1
  Mux2/1 -> Data Type Conversion21/1
  Data Type Conversion21/1 -> Out2/1
  Data Type Conversion22/1 -> Out1/1

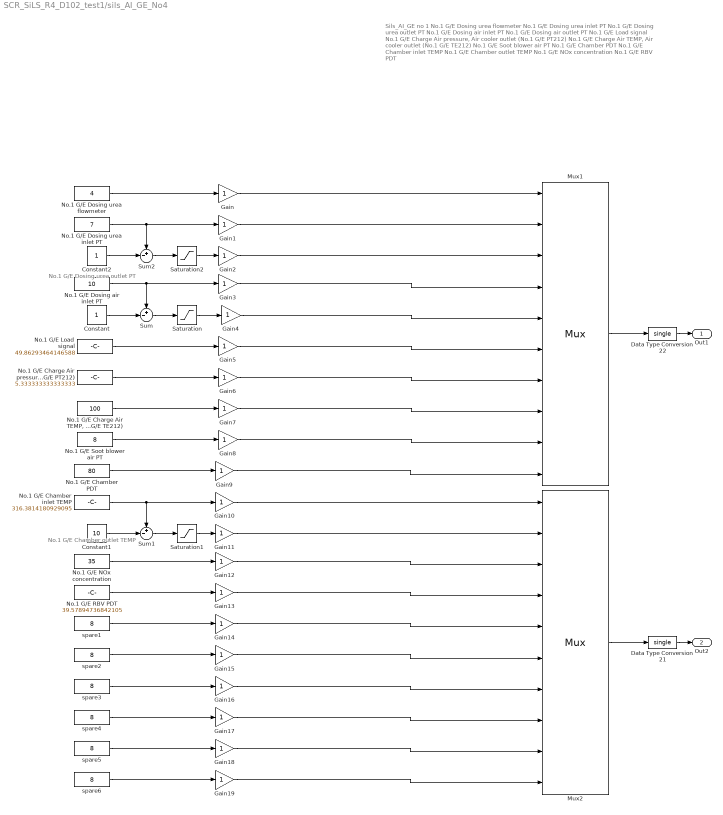
== system SCR_SiLS_R4_D102_test1/sils_AI_GE_No4 ==
  note: No.1 G/E Dosing urea outlet PT
  note: No.1 G/E Chamber outlet TEMP
  note: Sils_AI_GE no 1
      |
      | No.1 G/E Dosing urea flowmeter
      |
      | No.1 G/E Dosing urea inlet PT
      |
      | No.1 G/E Dosing urea outlet PT
      |
      | No.1 G/E Dosing air inlet PT
      |
      | No.1 G/E Dosing air outlet PT
      |
      | No.1 G/E Load signal
      |
      | No.1 G/E Charge Air pressure, Air cooler outlet (No.1 G/E PT212)
      |
      | No.1 G/E Charge Air TEMP, Air cooler outlet (No.1 G/E TE212)
      |
      | No.1 G/E Soot blower air PT
      |
      | No.1 G/E Chamber PDT
      |
      | No.1 G/E Chamber inlet TEMP
      |
      | No.1 G/E Chamber outlet TEMP
      |
      | No.1 G/E NOx concentration
      |
      | No.1 G/E RBV PDT
      |
      | ​
      |
      | ​
  Constant : Constant
  Constant1 : Constant  Value=10
  Constant2 : Constant
  Data Type Conversion21 : DataTypeConversion  OutDataTypeStr=single  SaturateOnIntegerOverflow=off  RndMeth=Floor
  Data Type Conversion22 : DataTypeConversion  OutDataTypeStr=single  SaturateOnIntegerOverflow=off  RndMeth=Floor
  Gain{,1..19} (20 alike) : Gain
  Mux1 : Mux  Inputs=10
  Mux2 : Mux  Inputs=10
  No.1 G/E Chamber PDT : Constant  Value=80
  No.1 G/E Chamber inlet TEMP : Constant  Value=316.3814180929095
  "No.1 G/E Charge Air TEMP, Air cooler outlet (No.1 G/E TE212)" : Constant  Value=100
  "No.1 G/E Charge Air pressure, Air cooler outlet (No.1 G/E PT212)" : Constant  Value=5.333333333333333
  No.1 G/E Dosing air inlet PT : Constant  Value=10
  No.1 G/E Dosing urea flowmeter : Constant  Value=4
  No.1 G/E Dosing urea inlet PT : Constant  Value=7
  No.1 G/E Load signal : Constant  Value=49.86293464146588
  No.1 G/E NOx concentration : Constant  Value=35
  No.1 G/E RBV PDT : Constant  Value=39.57894736842105
  No.1 G/E Soot blower air PT : Constant  Value=8
  Saturation : Saturate  UpperLimit=10.0  LowerLimit=0.0
  Saturation1 : Saturate  UpperLimit=500.0  LowerLimit=0.0
  Saturation2 : Saturate  UpperLimit=10.0  LowerLimit=0.0
  Sum : Sum  Inputs=+-|
  Sum1 : Sum  Inputs=+-|
  Sum2 : Sum  Inputs=+-|
  spare{1..6} (6 alike) : Constant  Value=8
  Out1 : Outport
  Out2 : Outport  Port=2
  wires:
  No.1 G/E Dosing urea flowmeter/1 -> Gain/1
  Gain1/1 -> Mux1/2
  Gain/1 -> Mux1/1
  Gain2/1 -> Mux1/3
  No.1 G/E Dosing air inlet PT/1 -> Gain3/1, Sum/1
  Sum/1 -> Saturation/1
  No.1 G/E Load signal/1 -> Gain5/1
  Gain3/1 -> Mux1/4
  Gain4/1 -> Mux1/5
  Gain5/1 -> Mux1/6
  "No.1 G/E Charge Air pressure, Air cooler outlet (No.1 G/E PT212)"/1 -> Gain6/1
  "No.1 G/E Charge Air TEMP, Air cooler outlet (No.1 G/E TE212)"/1 -> Gain7/1
  No.1 G/E Soot blower air PT/1 -> Gain8/1
  Gain6/1 -> Mux1/7
  Gain7/1 -> Mux1/8
  Gain8/1 -> Mux1/9
  No.1 G/E Chamber PDT/1 -> Gain9/1
  No.1 G/E Chamber inlet TEMP/1 -> Sum1/1, Gain10/1
  Gain9/1 -> Mux1/10
  Gain10/1 -> Mux2/1
  Gain11/1 -> Mux2/2
  No.1 G/E RBV PDT/1 -> Gain13/1
  Gain13/1 -> Mux2/4
  Gain12/1 -> Mux2/3
  No.1 G/E NOx concentration/1 -> Gain12/1
  Constant/1 -> Sum/2
  Saturation/1 -> Gain4/1
  Sum1/1 -> Saturation1/1
  Constant1/1 -> Sum1/2
  Saturation1/1 -> Gain11/1
  No.1 G/E Dosing urea inlet PT/1 -> Gain1/1, Sum2/1
  Sum2/1 -> Saturation2/1
  Constant2/1 -> Sum2/2
  Saturation2/1 -> Gain2/1
  spare1/1 -> Gain14/1
  Gain14/1 -> Mux2/5
  spare2/1 -> Gain15/1
  Gain15/1 -> Mux2/6
  spare3/1 -> Gain16/1
  Gain16/1 -> Mux2/7
  spare4/1 -> Gain17/1
  Gain17/1 -> Mux2/8
  spare5/1 -> Gain18/1
  Gain18/1 -> Mux2/9
  spare6/1 -> Gain19/1
  Gain19/1 -> Mux2/10
  Mux1/1 -> Data Type Conversion22/1
  Mux2/1 -> Data Type Conversion21/1
  Data Type Conversion21/1 -> Out2/1
  Data Type Conversion22/1 -> Out1/1

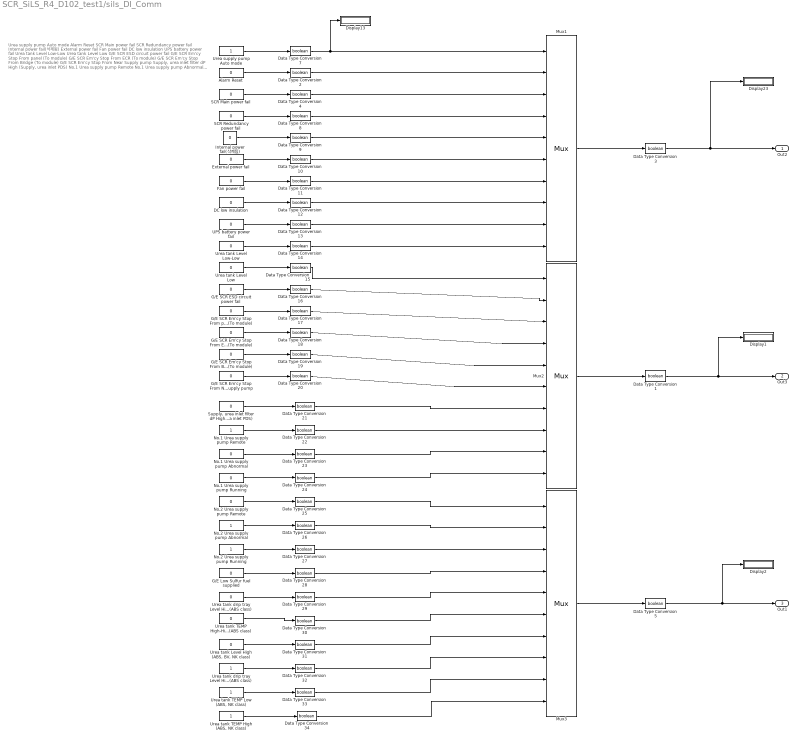
== system SCR_SiLS_R4_D102_test1/sils_DI_Comm ==
  note: Urea supply pump Auto mode
      |
      | Alarm Reset
      |
      | SCR Main power fail
      |
      | SCR Redundancy power fail
      |
      | Internal power fail(삭제됨)
      |
      | External power fail
      |
      | Fan power fail
      |
      | DC low insulation
      |
      | UPS battery power fail
      |
      | Urea tank Level Low-Low
      |
      | Urea tank Level Low
      |
      | G/E SCR ESD circuit power fail
      |
      | G/E SCR Em'cy Stop From panel (To module)
      |
      | G/E SCR Em'cy Stop From ECR (To module)
      |
      | G/E SCR Em'cy Stop From Bridge (To module)
      |
      | G/E SCR Em'cy Stop From Near Supply pump
      |
      | Supply, urea inlet filter dP High (Supply, urea inlet PDS)
      |
      | No.1 Urea supply pump Remote
      |
      | No.1 Urea supply pump Abnormal
      |
      | No.1 Urea supply pump Running
      |
      | No.2 Urea supply pump Remote
      |
      | No.2 Urea supply pump Abnormal
      |
      | No.2 Urea supply pump Running
      |
      | G/E Low Sulfur fuel supplied
      |
      | Urea tank drip tray Level High-High (ABS class)
      |
      | Urea tank TEMP High-High (ABS class)
      |
      | Urea tank Level High (ABS, BV, NK class)
      |
      | Urea tank drip tray Level High (ABS class)
      |
      | Urea tank TEMP Low (ABS, NK class)
      |
      | Urea tank TEMP High (ABS, NK class)
      |
      | ​
      |
      | ​
  Alarm Reset : Constant  Value=0
  DC low insulation : Constant  Value=0
  Data Type Conversion{1..5,7..34} (33 alike) : DataTypeConversion  OutDataTypeStr=boolean  SaturateOnIntegerOverflow=off  RndMeth=Floor
  Display{1..2,13,23} (4 alike) : Display
  External power fail : Constant  Value=0
  Fan power fail : Constant  Value=0
  G/E Low Sulfur fuel supplied : Constant  Value=0
  G/E SCR ESD circuit power fail : Constant  Value=0
  G/E SCR Em'cy Stop From Bridge (To module) : Constant  Value=0
  G/E SCR Em'cy Stop From ECR (To module) : Constant  Value=0
  G/E SCR Em'cy Stop From Near Supply pump : Constant  Value=0
  G/E SCR Em'cy Stop From panel (To module) : Constant  Value=0
  Internal power fail(삭제됨) : Constant  Value=0
  Mux1 : Mux  Inputs=10
  Mux2 : Mux  Inputs=10
  Mux3 : Mux  Inputs=10
  No.1 Urea supply pump Abnormal : Constant  Value=0
  No.1 Urea supply pump Remote : Constant
  No.1 Urea supply pump Running : Constant  Value=0
  No.2 Urea supply pump Abnormal : Constant
  No.2 Urea supply pump Remote : Constant  Value=0
  No.2 Urea supply pump Running : Constant
  SCR Main power fail : Constant  Value=0
  SCR Redundancy power fail : Constant  Value=0
  "Supply, urea inlet filter dP High (Supply, urea inlet PDS)" : Constant  Value=0
  UPS battery power fail : Constant  Value=0
  Urea supply pump Auto mode : Constant
  "Urea tank Level High (ABS, BV, NK class)" : Constant  Value=0
  Urea tank Level Low : Constant  Value=0
  Urea tank Level Low-Low : Constant  Value=0
  "Urea tank TEMP High (ABS, NK class)" : Constant
  Urea tank TEMP High-High (ABS class) : Constant  Value=0
  "Urea tank TEMP Low (ABS, NK class)" : Constant
  Urea tank drip tray Level High (ABS class) : Constant
  Urea tank drip tray Level High-High (ABS class) : Constant  Value=0
  Out2 : Outport
  Out3 : Outport  Port=2
  Out1 : Outport  Port=3
  wires:
  Urea supply pump Auto mode/1 -> Data Type Conversion7/1
  Data Type Conversion7/1 -> Display13/1, Mux1/1
  Data Type Conversion3/1 -> Display23/1, Out2/1
  Mux1/1 -> Data Type Conversion3/1
  Alarm Reset/1 -> Data Type Conversion2/1
  SCR Main power fail/1 -> Data Type Conversion4/1
  SCR Redundancy power fail/1 -> Data Type Conversion8/1
  Internal power fail(삭제됨)/1 -> Data Type Conversion9/1
  External power fail/1 -> Data Type Conversion10/1
  Fan power fail/1 -> Data Type Conversion11/1
  DC low insulation/1 -> Data Type Conversion12/1
  UPS battery power fail/1 -> Data Type Conversion13/1
  Urea tank Level Low-Low/1 -> Data Type Conversion14/1
  Urea tank Level Low/1 -> Data Type Conversion15/1
  G/E SCR ESD circuit power fail/1 -> Data Type Conversion16/1
  G/E SCR Em'cy Stop From panel (To module)/1 -> Data Type Conversion17/1
  G/E SCR Em'cy Stop From ECR (To module)/1 -> Data Type Conversion18/1
  G/E SCR Em'cy Stop From Bridge (To module)/1 -> Data Type Conversion19/1
  G/E SCR Em'cy Stop From Near Supply pump/1 -> Data Type Conversion20/1
  "Supply, urea inlet filter dP High (Supply, urea inlet PDS)"/1 -> Data Type Conversion21/1
  No.1 Urea supply pump Remote/1 -> Data Type Conversion22/1
  No.1 Urea supply pump Abnormal/1 -> Data Type Conversion23/1
  No.1 Urea supply pump Running/1 -> Data Type Conversion24/1
  No.2 Urea supply pump Remote/1 -> Data Type Conversion25/1
  No.2 Urea supply pump Abnormal/1 -> Data Type Conversion26/1
  No.2 Urea supply pump Running/1 -> Data Type Conversion27/1
  G/E Low Sulfur fuel supplied/1 -> Data Type Conversion28/1
  Urea tank drip tray Level High-High (ABS class)/1 -> Data Type Conversion29/1
  Urea tank TEMP High-High (ABS class)/1 -> Data Type Conversion30/1
  "Urea tank Level High (ABS, BV, NK class)"/1 -> Data Type Conversion31/1
  Urea tank drip tray Level High (ABS class)/1 -> Data Type Conversion32/1
  "Urea tank TEMP Low (ABS, NK class)"/1 -> Data Type Conversion33/1
  "Urea tank TEMP High (ABS, NK class)"/1 -> Data Type Conversion34/1
  Data Type Conversion2/1 -> Mux1/2
  Data Type Conversion4/1 -> Mux1/3
  Data Type Conversion8/1 -> Mux1/4
  Data Type Conversion9/1 -> Mux1/5
  Data Type Conversion10/1 -> Mux1/6
  Data Type Conversion11/1 -> Mux1/7
  Data Type Conversion12/1 -> Mux1/8
  Data Type Conversion13/1 -> Mux1/9
  Data Type Conversion14/1 -> Mux1/10
  Data Type Conversion15/1 -> Mux2/1
  Data Type Conversion16/1 -> Mux2/2
  Data Type Conversion17/1 -> Mux2/3
  Data Type Conversion18/1 -> Mux2/4
  Data Type Conversion19/1 -> Mux2/5
  Data Type Conversion20/1 -> Mux2/6
  Data Type Conversion21/1 -> Mux2/7
  Data Type Conversion25/1 -> Mux3/1
  Data Type Conversion22/1 -> Mux2/8
  Data Type Conversion23/1 -> Mux2/9
  Data Type Conversion24/1 -> Mux2/10
  Data Type Conversion28/1 -> Mux3/4
  Data Type Conversion27/1 -> Mux3/3
  Data Type Conversion26/1 -> Mux3/2
  Data Type Conversion29/1 -> Mux3/5
  Data Type Conversion32/1 -> Mux3/8
  Data Type Conversion31/1 -> Mux3/7
  Data Type Conversion30/1 -> Mux3/6
  Data Type Conversion33/1 -> Mux3/9
  Data Type Conversion34/1 -> Mux3/10
  Mux3/1 -> Data Type Conversion5/1
  Data Type Conversion5/1 -> Display2/1, Out1/1
  Mux2/1 -> Data Type Conversion1/1
  Data Type Conversion1/1 -> Display1/1, Out3/1

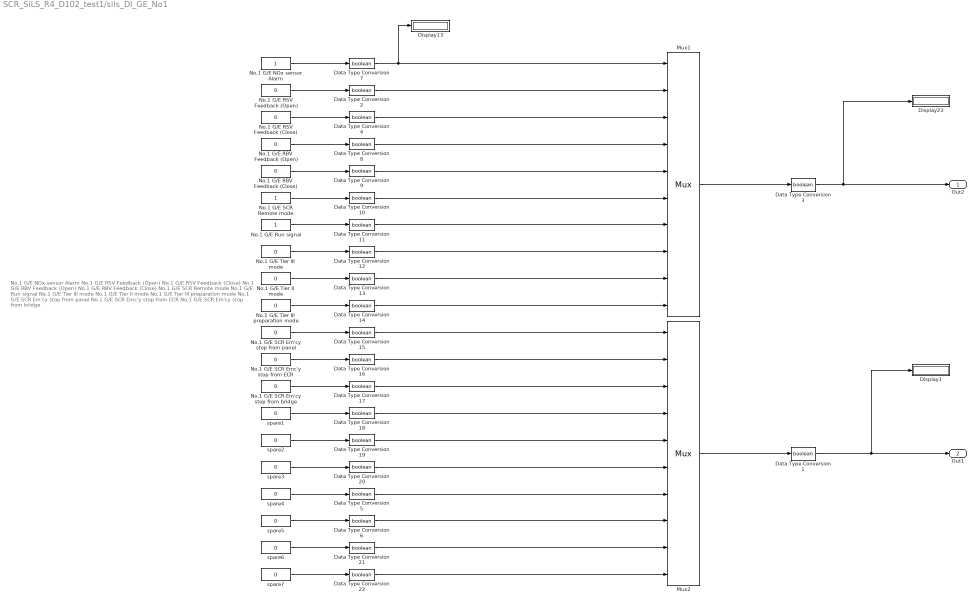
== system SCR_SiLS_R4_D102_test1/sils_DI_GE_No1 ==
  note: No.1 G/E NOx sensor Alarm
      |
      | No.1 G/E RSV Feedback (Open)
      |
      | No.1 G/E RSV Feedback (Close)
      |
      | No.1 G/E RBV Feedback (Open)
      |
      | No.1 G/E RBV Feedback (Close)
      |
      | No.1 G/E SCR Remote mode
      |
      | No.1 G/E Run signal
      |
      | No.1 G/E Tier III mode
      |
      | No.1 G/E Tier II mode
      |
      | No.1 G/E Tier III preparation mode
      |
      | No.1 G/E SCR Em'cy stop from panel
      |
      | No.1 G/E SCR Emc'y stop from ECR
      |
      | No.1 G/E SCR Em'cy stop from bridge
  Data Type Conversion{1..22} (22 alike) : DataTypeConversion  OutDataTypeStr=boolean  SaturateOnIntegerOverflow=off  RndMeth=Floor
  Display1 : Display
  Display13 : Display
  Display23 : Display
  Mux1 : Mux  Inputs=10
  Mux2 : Mux  Inputs=10
  No.1 G/E NOx sensor Alarm : Constant
  No.1 G/E RBV Feedback (Close) : Constant  Value=0
  No.1 G/E RBV Feedback (Open) : Constant  Value=0
  No.1 G/E RSV Feedback (Close) : Constant  Value=0
  No.1 G/E RSV Feedback (Open) : Constant  Value=0
  No.1 G/E Run signal : Constant
  No.1 G/E SCR Em'cy stop from bridge : Constant  Value=0
  No.1 G/E SCR Em'cy stop from panel : Constant  Value=0
  No.1 G/E SCR Emc'y stop from ECR : Constant  Value=0
  No.1 G/E SCR Remote mode : Constant
  No.1 G/E Tier II mode : Constant  Value=0
  No.1 G/E Tier III mode : Constant  Value=0
  No.1 G/E Tier III preparation mode : Constant  Value=0
  spare{1..7} (7 alike) : Constant  Value=0
  Out2 : Outport
  Out1 : Outport  Port=2
  wires:
  No.1 G/E NOx sensor Alarm/1 -> Data Type Conversion7/1
  Data Type Conversion7/1 -> Display13/1, Mux1/1
  Data Type Conversion3/1 -> Out2/1, Display23/1
  Mux1/1 -> Data Type Conversion3/1
  No.1 G/E RSV Feedback (Open)/1 -> Data Type Conversion2/1
  No.1 G/E RSV Feedback (Close)/1 -> Data Type Conversion4/1
  No.1 G/E RBV Feedback (Open)/1 -> Data Type Conversion8/1
  No.1 G/E RBV Feedback (Close)/1 -> Data Type Conversion9/1
  No.1 G/E SCR Remote mode/1 -> Data Type Conversion10/1
  No.1 G/E Run signal/1 -> Data Type Conversion11/1
  No.1 G/E Tier III mode/1 -> Data Type Conversion12/1
  No.1 G/E Tier II mode/1 -> Data Type Conversion13/1
  No.1 G/E Tier III preparation mode/1 -> Data Type Conversion14/1
  No.1 G/E SCR Em'cy stop from panel/1 -> Data Type Conversion15/1
  No.1 G/E SCR Emc'y stop from ECR/1 -> Data Type Conversion16/1
  No.1 G/E SCR Em'cy stop from bridge/1 -> Data Type Conversion17/1
  spare1/1 -> Data Type Conversion18/1
  spare2/1 -> Data Type Conversion19/1
  spare3/1 -> Data Type Conversion20/1
  Data Type Conversion2/1 -> Mux1/2
  Data Type Conversion4/1 -> Mux1/3
  Data Type Conversion8/1 -> Mux1/4
  Data Type Conversion9/1 -> Mux1/5
  Data Type Conversion10/1 -> Mux1/6
  Data Type Conversion11/1 -> Mux1/7
  Data Type Conversion12/1 -> Mux1/8
  Data Type Conversion13/1 -> Mux1/9
  Data Type Conversion14/1 -> Mux1/10
  Data Type Conversion15/1 -> Mux2/1
  Data Type Conversion16/1 -> Mux2/2
  Data Type Conversion17/1 -> Mux2/3
  Data Type Conversion18/1 -> Mux2/4
  Data Type Conversion19/1 -> Mux2/5
  Data Type Conversion20/1 -> Mux2/6
  Data Type Conversion1/1 -> Out1/1, Display1/1
  Mux2/1 -> Data Type Conversion1/1
  spare4/1 -> Data Type Conversion5/1
  spare5/1 -> Data Type Conversion6/1
  Data Type Conversion5/1 -> Mux2/7
  Data Type Conversion6/1 -> Mux2/8
  spare6/1 -> Data Type Conversion21/1
  spare7/1 -> Data Type Conversion22/1
  Data Type Conversion21/1 -> Mux2/9
  Data Type Conversion22/1 -> Mux2/10

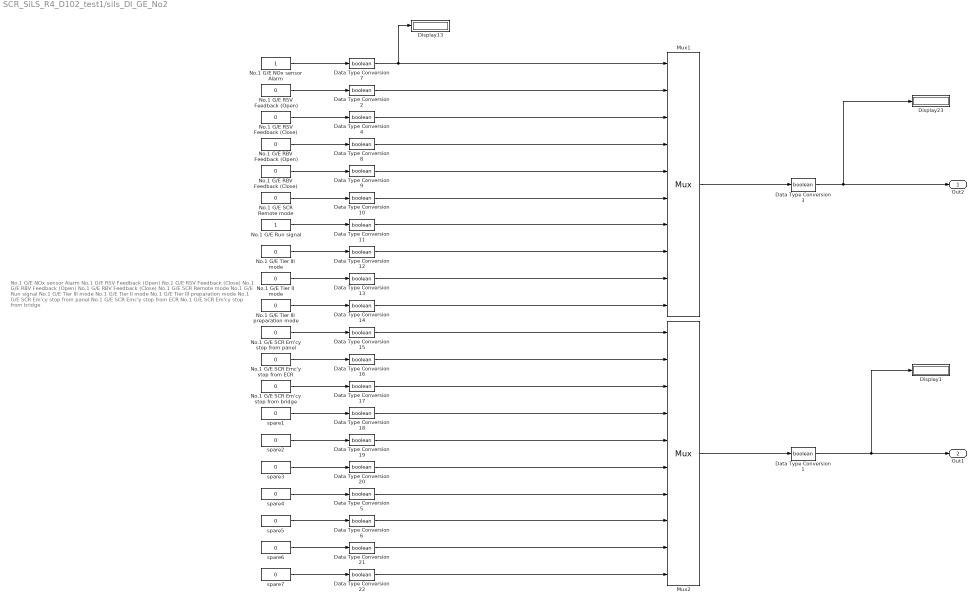
== system SCR_SiLS_R4_D102_test1/sils_DI_GE_No2 ==
  note: No.1 G/E NOx sensor Alarm
      |
      | No.1 G/E RSV Feedback (Open)
      |
      | No.1 G/E RSV Feedback (Close)
      |
      | No.1 G/E RBV Feedback (Open)
      |
      | No.1 G/E RBV Feedback (Close)
      |
      | No.1 G/E SCR Remote mode
      |
      | No.1 G/E Run signal
      |
      | No.1 G/E Tier III mode
      |
      | No.1 G/E Tier II mode
      |
      | No.1 G/E Tier III preparation mode
      |
      | No.1 G/E SCR Em'cy stop from panel
      |
      | No.1 G/E SCR Emc'y stop from ECR
      |
      | No.1 G/E SCR Em'cy stop from bridge
  Data Type Conversion{1..22} (22 alike) : DataTypeConversion  OutDataTypeStr=boolean  SaturateOnIntegerOverflow=off  RndMeth=Floor
  Display1 : Display
  Display13 : Display
  Display23 : Display
  Mux1 : Mux  Inputs=10
  Mux2 : Mux  Inputs=10
  No.1 G/E NOx sensor Alarm : Constant
  No.1 G/E RBV Feedback (Close) : Constant  Value=0
  No.1 G/E RBV Feedback (Open) : Constant  Value=0
  No.1 G/E RSV Feedback (Close) : Constant  Value=0
  No.1 G/E RSV Feedback (Open) : Constant  Value=0
  No.1 G/E Run signal : Constant
  No.1 G/E SCR Em'cy stop from bridge : Constant  Value=0
  No.1 G/E SCR Em'cy stop from panel : Constant  Value=0
  No.1 G/E SCR Emc'y stop from ECR : Constant  Value=0
  No.1 G/E SCR Remote mode : Constant  Value=0
  No.1 G/E Tier II mode : Constant  Value=0
  No.1 G/E Tier III mode : Constant  Value=0
  No.1 G/E Tier III preparation mode : Constant  Value=0
  spare{1..7} (7 alike) : Constant  Value=0
  Out2 : Outport
  Out1 : Outport  Port=2
  wires:
  No.1 G/E NOx sensor Alarm/1 -> Data Type Conversion7/1
  Data Type Conversion7/1 -> Display13/1, Mux1/1
  Data Type Conversion3/1 -> Out2/1, Display23/1
  Mux1/1 -> Data Type Conversion3/1
  No.1 G/E RSV Feedback (Open)/1 -> Data Type Conversion2/1
  No.1 G/E RSV Feedback (Close)/1 -> Data Type Conversion4/1
  No.1 G/E RBV Feedback (Open)/1 -> Data Type Conversion8/1
  No.1 G/E RBV Feedback (Close)/1 -> Data Type Conversion9/1
  No.1 G/E SCR Remote mode/1 -> Data Type Conversion10/1
  No.1 G/E Run signal/1 -> Data Type Conversion11/1
  No.1 G/E Tier III mode/1 -> Data Type Conversion12/1
  No.1 G/E Tier II mode/1 -> Data Type Conversion13/1
  No.1 G/E Tier III preparation mode/1 -> Data Type Conversion14/1
  No.1 G/E SCR Em'cy stop from panel/1 -> Data Type Conversion15/1
  No.1 G/E SCR Emc'y stop from ECR/1 -> Data Type Conversion16/1
  No.1 G/E SCR Em'cy stop from bridge/1 -> Data Type Conversion17/1
  spare1/1 -> Data Type Conversion18/1
  spare2/1 -> Data Type Conversion19/1
  spare3/1 -> Data Type Conversion20/1
  Data Type Conversion2/1 -> Mux1/2
  Data Type Conversion4/1 -> Mux1/3
  Data Type Conversion8/1 -> Mux1/4
  Data Type Conversion9/1 -> Mux1/5
  Data Type Conversion10/1 -> Mux1/6
  Data Type Conversion11/1 -> Mux1/7
  Data Type Conversion12/1 -> Mux1/8
  Data Type Conversion13/1 -> Mux1/9
  Data Type Conversion14/1 -> Mux1/10
  Data Type Conversion15/1 -> Mux2/1
  Data Type Conversion16/1 -> Mux2/2
  Data Type Conversion17/1 -> Mux2/3
  Data Type Conversion18/1 -> Mux2/4
  Data Type Conversion19/1 -> Mux2/5
  Data Type Conversion20/1 -> Mux2/6
  Data Type Conversion1/1 -> Out1/1, Display1/1
  Mux2/1 -> Data Type Conversion1/1
  spare4/1 -> Data Type Conversion5/1
  spare5/1 -> Data Type Conversion6/1
  Data Type Conversion5/1 -> Mux2/7
  Data Type Conversion6/1 -> Mux2/8
  spare6/1 -> Data Type Conversion21/1
  spare7/1 -> Data Type Conversion22/1
  Data Type Conversion21/1 -> Mux2/9
  Data Type Conversion22/1 -> Mux2/10

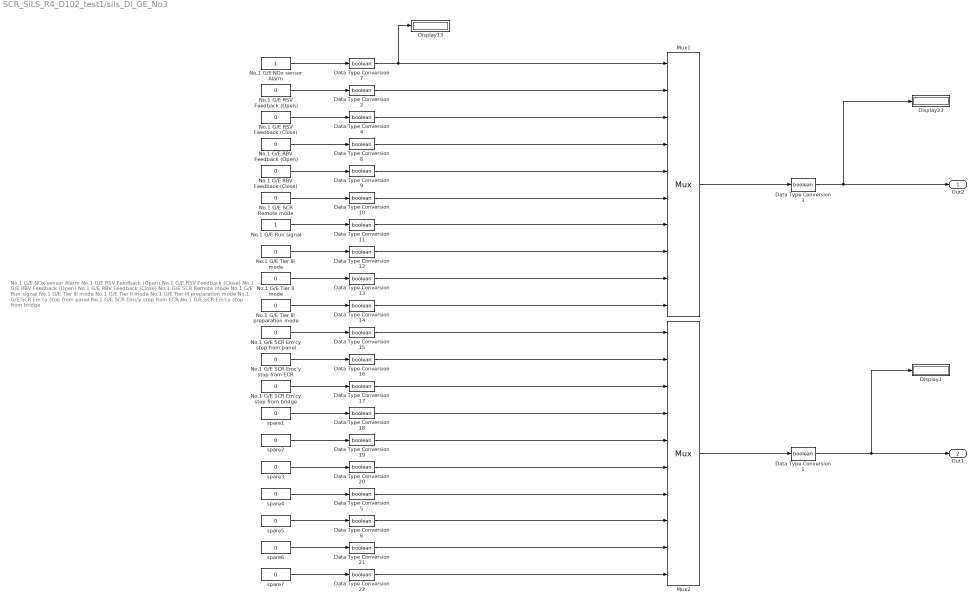
== system SCR_SiLS_R4_D102_test1/sils_DI_GE_No3 ==
  note: No.1 G/E NOx sensor Alarm
      |
      | No.1 G/E RSV Feedback (Open)
      |
      | No.1 G/E RSV Feedback (Close)
      |
      | No.1 G/E RBV Feedback (Open)
      |
      | No.1 G/E RBV Feedback (Close)
      |
      | No.1 G/E SCR Remote mode
      |
      | No.1 G/E Run signal
      |
      | No.1 G/E Tier III mode
      |
      | No.1 G/E Tier II mode
      |
      | No.1 G/E Tier III preparation mode
      |
      | No.1 G/E SCR Em'cy stop from panel
      |
      | No.1 G/E SCR Emc'y stop from ECR
      |
      | No.1 G/E SCR Em'cy stop from bridge
  Data Type Conversion{1..22} (22 alike) : DataTypeConversion  OutDataTypeStr=boolean  SaturateOnIntegerOverflow=off  RndMeth=Floor
  Display1 : Display
  Display13 : Display
  Display23 : Display
  Mux1 : Mux  Inputs=10
  Mux2 : Mux  Inputs=10
  No.1 G/E NOx sensor Alarm : Constant
  No.1 G/E RBV Feedback (Close) : Constant  Value=0
  No.1 G/E RBV Feedback (Open) : Constant  Value=0
  No.1 G/E RSV Feedback (Close) : Constant  Value=0
  No.1 G/E RSV Feedback (Open) : Constant  Value=0
  No.1 G/E Run signal : Constant
  No.1 G/E SCR Em'cy stop from bridge : Constant  Value=0
  No.1 G/E SCR Em'cy stop from panel : Constant  Value=0
  No.1 G/E SCR Emc'y stop from ECR : Constant  Value=0
  No.1 G/E SCR Remote mode : Constant  Value=0
  No.1 G/E Tier II mode : Constant  Value=0
  No.1 G/E Tier III mode : Constant  Value=0
  No.1 G/E Tier III preparation mode : Constant  Value=0
  spare{1..7} (7 alike) : Constant  Value=0
  Out2 : Outport
  Out1 : Outport  Port=2
  wires:
  No.1 G/E NOx sensor Alarm/1 -> Data Type Conversion7/1
  Data Type Conversion7/1 -> Display13/1, Mux1/1
  Data Type Conversion3/1 -> Out2/1, Display23/1
  Mux1/1 -> Data Type Conversion3/1
  No.1 G/E RSV Feedback (Open)/1 -> Data Type Conversion2/1
  No.1 G/E RSV Feedback (Close)/1 -> Data Type Conversion4/1
  No.1 G/E RBV Feedback (Open)/1 -> Data Type Conversion8/1
  No.1 G/E RBV Feedback (Close)/1 -> Data Type Conversion9/1
  No.1 G/E SCR Remote mode/1 -> Data Type Conversion10/1
  No.1 G/E Run signal/1 -> Data Type Conversion11/1
  No.1 G/E Tier III mode/1 -> Data Type Conversion12/1
  No.1 G/E Tier II mode/1 -> Data Type Conversion13/1
  No.1 G/E Tier III preparation mode/1 -> Data Type Conversion14/1
  No.1 G/E SCR Em'cy stop from panel/1 -> Data Type Conversion15/1
  No.1 G/E SCR Emc'y stop from ECR/1 -> Data Type Conversion16/1
  No.1 G/E SCR Em'cy stop from bridge/1 -> Data Type Conversion17/1
  spare1/1 -> Data Type Conversion18/1
  spare2/1 -> Data Type Conversion19/1
  spare3/1 -> Data Type Conversion20/1
  Data Type Conversion2/1 -> Mux1/2
  Data Type Conversion4/1 -> Mux1/3
  Data Type Conversion8/1 -> Mux1/4
  Data Type Conversion9/1 -> Mux1/5
  Data Type Conversion10/1 -> Mux1/6
  Data Type Conversion11/1 -> Mux1/7
  Data Type Conversion12/1 -> Mux1/8
  Data Type Conversion13/1 -> Mux1/9
  Data Type Conversion14/1 -> Mux1/10
  Data Type Conversion15/1 -> Mux2/1
  Data Type Conversion16/1 -> Mux2/2
  Data Type Conversion17/1 -> Mux2/3
  Data Type Conversion18/1 -> Mux2/4
  Data Type Conversion19/1 -> Mux2/5
  Data Type Conversion20/1 -> Mux2/6
  Data Type Conversion1/1 -> Out1/1, Display1/1
  Mux2/1 -> Data Type Conversion1/1
  spare4/1 -> Data Type Conversion5/1
  spare5/1 -> Data Type Conversion6/1
  Data Type Conversion5/1 -> Mux2/7
  Data Type Conversion6/1 -> Mux2/8
  spare6/1 -> Data Type Conversion21/1
  spare7/1 -> Data Type Conversion22/1
  Data Type Conversion21/1 -> Mux2/9
  Data Type Conversion22/1 -> Mux2/10
